simulink model "InnerOuter_Sim"  (Simulink 6.6)
settings: Solver=ode4  StartTime=0.0  StopTime=700  FixedStep=SampleT  RelTol=1e-3
InitFcn:
  | clc
  | Rascal_Var
  | innerOuterInit
  | wpFile
values from neighbouring files (symbols this model uses):
  A1 = 0.007    [Rascal_Var.m]
  Apolar = 0.057    [Rascal_Var.m]
  apSampleTime = 0.01    [innerOuterInit.m]
  CD0 = 0.022    [Rascal_Var.m]
  chord = S/span    (= 0.351341681574)    [Rascal_Var.m]
  CL0 = 0.38    [Rascal_Var.m]
  CLa = 18.5    [Rascal_Var.m]
  CLa_dot = 2.64    [Rascal_Var.m]
  Clb = -0.296    [Rascal_Var.m]
  ClDa = 0.1695    [Rascal_Var.m]
  CLDe = 0.24    [Rascal_Var.m]
  CLDf = 0.4    [Rascal_Var.m]
  ClDr = 0.106    [Rascal_Var.m]
  Clp = -1.96    [Rascal_Var.m]
  CLq = 7.4    [Rascal_Var.m]
  Clr = 0.103    [Rascal_Var.m]
  Cm0 = 0.3    [Rascal_Var.m]
  Cma = -1.239    [Rascal_Var.m]
  CmDe = -3.2    [Rascal_Var.m]
  CmDf = -.021    (= -0.021)    [Rascal_Var.m]
  Cmq = -2.4    [Rascal_Var.m]
  Cnb = 0.277    [Rascal_Var.m]
  CnDa = -0.023    [Rascal_Var.m]
  CnDr = -0.1997    [Rascal_Var.m]
  Cnp = -0.0889    [Rascal_Var.m]
  Cnr = -0.19997    [Rascal_Var.m]
  CYb = -1.098    [Rascal_Var.m]
  CYDr = 0.143    [Rascal_Var.m]
  derivativesConstant = 5    [innerOuterInit.m]
  elarm = 1.21    [Rascal_Var.m]
  Euler_0 = [0; 0; 90*pi/180]'    [Rascal_Var.m]    (also in randomInit.m = double([0; 0; psi_ic]'))
  ISA_g = 9.815    [Rascal_Var.m]
  Ixx = 4.12    [Rascal_Var.m]
  Iyy = 9.58    [Rascal_Var.m]
  Izz = 9.85    [Rascal_Var.m]
  mass = 0.45359237*18    (= 8.16466266)    [Rascal_Var.m]
  MinThK = 0.077    [Rascal_Var.m]
  Pos_0 = [0; 0 ;450]'    [Rascal_Var.m]    (also in randomInit.m = double([x_ic y_ic z_ic]))
  PQR_0 = [0;0;0]'    [Rascal_Var.m]
  SampleT = 0.005    [Rascal_Var.m]    (also in innerOuterInit.m)
  span = 2.795    [Rascal_Var.m]
  ThK = 2.17    [Rascal_Var.m]
  Vb_0 = [ 25; 0;0]'    [Rascal_Var.m]
  wpCount = uint8(floor(getRanVal(7,4,10)))    [randomInit.m]
undefined symbols (not defined in the file or in its folder): bankCommandLimit, clock, daLimit, deg, deLimit, DiscIntNeverNeededParam, drLimit, dtLimit, Earth, heightErrorLimit, pitchCommandLimit, pitchErrorLimit, rad, rollControlLimit, s, uHoldLimit, WGS84, yawDamperLimit
libraries: simulink x54, SLUGS_Library x14, aerolibconvert2 x9, aerolibtransform2 x2, aerolibwind2 x1, aerolibatmos2 x1, dspmtrx3 x1, dsPICdrivers x1
(part 2 of 2)

== system InnerOuter_Sim/6DOF Model/Plant/Engine Model/Get To1 ==
  dt : Inport
  Divide : Product  Inputs=3  OutScaling=2^-10
  Math Function : Math  Operator=pow  SaturateOnIntegerOverflow=on
  Math Function1 : Math  Operator=pow  SaturateOnIntegerOverflow=on
  MaxRPM : Gain  Gain=7200  SaturateOnIntegerOverflow=on
  Min RPM : Constant  Value=2000
  Min Th K : Constant  Value=MinThK
  Prop Diameter (in) : Constant  Value=17
  Prop Diameter (in)1 : Constant  Value=2
  Prop Diameter (in)2 : Constant  Value=4
  Saturation : Saturate  UpperLimit=1.0  LowerLimit=0.2
  Sum : Sum  Inputs=|++
  Sum1 : Sum  Inputs=|++
  TFact : simulink/Math Operations/Slider Gain  SystemSampleTime=-1  low=0  gain=0.2  high=1
  Th K : Gain  Gain=ThK  SaturateOnIntegerOverflow=on
  To Constant : Constant  Value=2.83e-12
  To : Outport
  wires:
  Saturation/1 -> Th K/1
  Prop Diameter (in)1/1 -> Math Function/2
  Prop Diameter (in)2/1 -> Math Function1/2
  Prop Diameter (in)/1 -> Math Function1/1
  Math Function/1 -> Divide/1
  Math Function1/1 -> Divide/2
  To Constant/1 -> Divide/3
  Divide/1 -> TFact/1
  TFact/1 -> To/1
  Sum/1 -> Math Function/1
  Min RPM/1 -> Sum/2
  MaxRPM/1 -> Sum/1
  Th K/1 -> Sum1/1
  dt/1 -> Saturation/1
  Sum1/1 -> MaxRPM/1
  Min Th K/1 -> Sum1/2

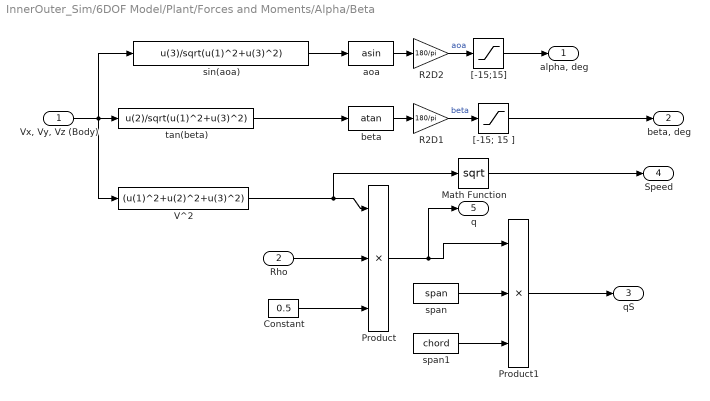
== system InnerOuter_Sim/6DOF Model/Plant/Forces and Moments/Alpha/Beta ==
  "Vx, Vy, Vz (Body)" : Inport
  Rho : Inport  Port=2
  Constant : Constant  Value=0.5  VectorParams1D=off
  Math Function : Math  Operator=sqrt  SaturateOnIntegerOverflow=on
  Product : Product  Inputs=3  SaturateOnIntegerOverflow=on
  Product1 : Product  Inputs=3  SaturateOnIntegerOverflow=on
  R2D1 : Gain  Gain=180/pi  SaturateOnIntegerOverflow=on
  R2D2 : Gain  Gain=180/pi  SaturateOnIntegerOverflow=on
  V^2 : Fcn  Expr=(u(1)^2+u(2)^2+u(3)^2)
  "[-15; 15 ]" : Saturate  UpperLimit=15  LowerLimit=-15
  "[-15;15]" : Saturate  UpperLimit=15  LowerLimit=-15
  aoa : Trigonometry  Operator=asin
  beta : Trigonometry  Operator=atan
  sin(aoa) : Fcn  Expr=u(3)/sqrt(u(1)^2+u(3)^2)
  span : Constant  Value=span  VectorParams1D=off
  span1 : Constant  Value=chord  VectorParams1D=off
  tan(beta) : Fcn  Expr=u(2)/sqrt(u(1)^2+u(3)^2)
  "alpha, deg" : Outport
  "beta, deg" : Outport  Port=2
  qS : Outport  Port=3
  Speed : Outport  Port=4
  q : Outport  Port=5
  wires:
  Product/1 -> q/1, Product1/1
  Product1/1 -> qS/1
  span1/1 -> Product1/3
  span/1 -> Product1/2
  "Vx, Vy, Vz (Body)"/1 -> sin(aoa)/1, V^2/1, tan(beta)/1
  tan(beta)/1 -> beta/1
  beta/1 -> R2D1/1
  V^2/1 -> Product/1, Math Function/1
  Rho/1 -> Product/2
  Constant/1 -> Product/3
  R2D1/1 -> "[-15; 15 ]"/1  "beta"
  aoa/1 -> R2D2/1
  R2D2/1 -> "[-15;15]"/1  "aoa"
  sin(aoa)/1 -> aoa/1
  Math Function/1 -> Speed/1
  "[-15;15]"/1 -> "alpha, deg"/1
  "[-15; 15 ]"/1 -> "beta, deg"/1

== system InnerOuter_Sim/6DOF Model/Plant/Forces and Moments/Body Frame F & M ==
  "Alpha, deg" : Inport
  "Beta, deg" : Inport  Port=2
  qs : Inport  Port=3
  Airspeed : Inport  Port=4
  "de, deg" : Inport  Port=5
  "da, deg" : Inport  Port=6
  "dr, deg" : Inport  Port=7
  "df, deg" : Inport  Port=8
  p,q,r : Inport  Port=9
  Bus Creator : BusCreator  Inputs=2
  Transfer to body frame : Subsystem
  Wind frame F& M : Subsystem
  F_b : Outport
  M_b : Outport  Port=2
  wires:
  "Alpha, deg"/1 -> Wind frame F& M/1("alpha, deg"), Bus Creator/1
  "Beta, deg"/1 -> Wind frame F& M/2("beta, deg"), Bus Creator/2
  "dr, deg"/1 -> Wind frame F& M/5("dr, deg")
  "da, deg"/1 -> Wind frame F& M/4("da, deg")
  "de, deg"/1 -> Wind frame F& M/3("de, deg")
  Wind frame F& M/1(F&M wind frame) -> Transfer to body frame/1(Wind frame  F&M)
  Bus Creator/1 -> Transfer to body frame/2("aoa/beta, deg")  "aoa/beta, deg"
  Transfer to body frame/1(F_b) -> F_b/1
  Transfer to body frame/2(M_b) -> M_b/1
  "df, deg"/1 -> Wind frame F& M/6("df, deg")
  qs/1 -> Wind frame F& M/7(qS)
  p,q,r/1 -> Wind frame F& M/8(p,q,r)
  Airspeed/1 -> Wind frame F& M/9(Airpseed)

== system InnerOuter_Sim/6DOF Model/Plant/Forces and Moments/Get Grav Force in Body ==
  Euler : Inport
  Grav Force : Inport  Port=2
  Math Function : Math  Operator=transpose  SaturateOnIntegerOverflow=on
  Product1 : Product  Multiplication=Matrix(*)  SaturateOnIntegerOverflow=on  InputSameDT=on
  Rb2u : Subsystem
  Reshape : Reshape  OutputDimensionality=Column vector (2-D)
  Grav Force (Body) : Outport
  wires:
  Rb2u/1(DCM) -> Math Function/1
  Euler/1 -> Rb2u/1(phi theta psi)
  Product1/1 -> Grav Force (Body)/1
  Math Function/1 -> Product1/1
  Grav Force/1 -> Reshape/1
  Reshape/1 -> Product1/2

== system InnerOuter_Sim/6DOF Model/Plant/Forces and Moments/NED(u)2b ==
  V w : Inport
  Euler : Inport  Port=2
  RB2LTP : Subsystem
  RL2B * Vw : Product  Multiplication=Matrix(*)  SaturateOnIntegerOverflow=on  InputSameDT=on
  RLTP2B : Math  Operator=transpose  SaturateOnIntegerOverflow=on
  Reshape1 : Reshape  OutputDimensionality=Row vector (2-D)
  Vb Corr : Outport
  wires:
  RL2B * Vw/1 -> Reshape1/1
  Euler/1 -> RB2LTP/1(Euler)
  RB2LTP/1(RB2L) -> RLTP2B/1
  RLTP2B/1 -> RL2B * Vw/1
  V w/1 -> RL2B * Vw/2
  Reshape1/1 -> Vb Corr/1

== system InnerOuter_Sim/6DOF Model/Plant/Magnetometer/RB2LTP ==
  Euler : Inport
  11 : Fcn  Expr=cos(u[3])*cos(u[2])
  12 : Fcn  Expr=sin(u[3])*cos(u[2])
  13 : Fcn  Expr=-sin(u[2])
  21 : Fcn  Expr=cos(u[3])*sin(u[2])*sin(u[1])-sin(u[3])*cos(u[1])
  22 : Fcn  Expr=sin(u[3])*sin(u[2])*sin(u[1])+cos(u[3])*cos(u[1])
  23 : Fcn  Expr=cos(u[2])*sin(u[1])
  31 : Fcn  Expr=cos(u[3])*sin(u[2])*cos(u[1])+sin(u[3])*sin(u[1])
  32 : Fcn  Expr=sin(u[3])*sin(u[2])*cos(u[1])-cos(u[3])*sin(u[1])
  33 : Fcn  Expr=cos(u[2])*cos(u[1])
  Mux2 : Mux  Inputs=9
  Reshape : Reshape  OutputDimensionality=Customize  OutputDimensions=[3,3]
  Rot : Outport
  wires:
  33/1 -> Mux2/9
  32/1 -> Mux2/8
  31/1 -> Mux2/7
  23/1 -> Mux2/6
  22/1 -> Mux2/5
  21/1 -> Mux2/4
  13/1 -> Mux2/3
  12/1 -> Mux2/2
  11/1 -> Mux2/1
  Mux2/1 -> Reshape/1
  Euler/1 -> 11/1, 33/1, 32/1, 31/1, 23/1, 22/1, 21/1, 13/1, 12/1
  Reshape/1 -> Rot/1

== system InnerOuter_Sim/6DOF Model/Plant/Wrap Around PSI1/Negative Yaw ==
  yaw : Inport
  Enable : EnablePort
  Abs : Abs
  Constant1 : Constant  Value=2*pi
  Constant2 : Constant  Value=2*pi
  Math Function : Math  Operator=mod  SaturateOnIntegerOverflow=on
  Sum : Sum  Inputs=|-+
  yaw_wr : Outport
  wires:
  yaw/1 -> Abs/1
  Constant1/1 -> Math Function/2
  Math Function/1 -> Sum/1
  Abs/1 -> Math Function/1
  Constant2/1 -> Sum/2
  Sum/1 -> yaw_wr/1

== system InnerOuter_Sim/6DOF Model/Plant/Wrap Around PSI1/Positive Yaw ==
  yaw : Inport
  Enable : EnablePort
  Constant1 : Constant  Value=2*pi
  Math Function : Math  Operator=mod  SaturateOnIntegerOverflow=on
  yaw_wr : Outport
  wires:
  yaw/1 -> Math Function/1
  Constant1/1 -> Math Function/2
  Math Function/1 -> yaw_wr/1

== system InnerOuter_Sim/6DOF Model/Plant/6-DOF EOM/[V1,2,3,W1,2,3]/A = [M ; J] ==
  Constant1 : Constant  Value=zeros(3,3)
  Constant4 : Constant  Value=0
  Display : Display
  Display1 : Display
  Display2 : Display
  Ixx : Constant  Value=Ixx  VectorParams1D=off
  Iyy : Constant  Value=Iyy  VectorParams1D=off
  Izz : Constant  Value=Izz  VectorParams1D=off
  Matrix Concatenation : Concatenate  Mode=Multidimensional array
  Matrix Concatenation1 : Concatenate  Mode=Multidimensional array
  Matrix Concatenation2 : Concatenate  Mode=Multidimensional array  ConcatenateDimension=2
  Mux : Mux  Inputs=9
  Mux1 : Mux  Inputs=9
  Reshape : Reshape  OutputDimensionality=Customize  OutputDimensions=[3,3]
  Reshape1 : Reshape  OutputDimensionality=Customize  OutputDimensions=[3,3]
  mass : Constant  Value=mass  VectorParams1D=off
  A Matrix : Outport
  wires:
  Ixx/1 -> Mux/1
  Izz/1 -> Mux/9
  Iyy/1 -> Mux/5
  Constant4/1 -> Mux/8, Mux/7, Mux/6, Mux/4, Mux/3, Mux/2, Mux1/8, Mux1/7, Mux1/6, Mux1/4, Mux1/3, Mux1/2
  mass/1 -> Mux1/1, Mux1/5, Mux1/9
  Mux1/1 -> Reshape/1
  Mux/1 -> Reshape1/1
  Matrix Concatenation/1 -> Matrix Concatenation2/1, Display/1
  Matrix Concatenation1/1 -> Matrix Concatenation2/2, Display1/1
  Matrix Concatenation2/1 -> A Matrix/1, Display2/1
  Reshape1/1 -> Matrix Concatenation1/2
  Reshape/1 -> Matrix Concatenation/1
  Constant1/1 -> Matrix Concatenation/2, Matrix Concatenation1/1

== system InnerOuter_Sim/6DOF Model/Plant/6-DOF EOM/[V1,2,3,W1,2,3]/Get Grav Force in Body ==
  Euler : Inport
  Grav Force : Inport  Port=2
  Math Function : Math  Operator=transpose  SaturateOnIntegerOverflow=on
  Product1 : Product  Multiplication=Matrix(*)  SaturateOnIntegerOverflow=on  InputSameDT=on
  Rb2u : Subsystem
  Reshape : Reshape  OutputDimensionality=Column vector (2-D)
  Grav Force (Body) : Outport
  wires:
  Rb2u/1(DCM) -> Math Function/1
  Euler/1 -> Rb2u/1(phi theta psi)
  Product1/1 -> Grav Force (Body)/1
  Math Function/1 -> Product1/1
  Grav Force/1 -> Reshape/1
  Reshape/1 -> Product1/2

== system InnerOuter_Sim/6DOF Model/Plant/6-DOF EOM/[V1,2,3,W1,2,3]/Sigma ==
  note: S(pqr)
  pqr : Inport
  Gain : Gain  Gain=[0 0 0;0 0 -1; 0 1 0]  Multiplication=Matrix(K*u)  SaturateOnIntegerOverflow=on
  Gain1 : Gain  Gain=[0 0 1;0 0 0; -1 0 0]  Multiplication=Matrix(K*u)  SaturateOnIntegerOverflow=on
  Gain2 : Gain  Gain="[0 -1 0;1 0 0;  0 0 0]"  Multiplication=Matrix(K*u)  SaturateOnIntegerOverflow=on
  Gain3 : Gain  Gain=0  SaturateOnIntegerOverflow=on
  Math Function : Math  Operator=transpose  SaturateOnIntegerOverflow=on
  Matrix Concatenation : Concatenate  Mode=Multidimensional array  ConcatenateDimension=2
  Matrix Concatenation1 : Concatenate  Mode=Multidimensional array  ConcatenateDimension=2
  Matrix Concatenation2 : Concatenate  Mode=Multidimensional array
  Mux : Mux  Inputs=3
  Reshape : Reshape  OutputDimensionality=Customize  OutputDimensions=[3,3]
  Sigma : Outport
  wires:
  Mux/1 -> Reshape/1
  Gain/1 -> Mux/1
  Gain1/1 -> Mux/2
  Gain2/1 -> Mux/3
  Reshape/1 -> Math Function/1
  Math Function/1 -> Gain3/1, Matrix Concatenation/1, Matrix Concatenation1/2
  Gain3/1 -> Matrix Concatenation/2, Matrix Concatenation1/1
  Matrix Concatenation/1 -> Matrix Concatenation2/1
  Matrix Concatenation1/1 -> Matrix Concatenation2/2
  Matrix Concatenation2/1 -> Sigma/1
  pqr/1 -> Gain/1, Gain2/1, Gain1/1

== system InnerOuter_Sim/6DOF Model/Plant/Forces and Moments/Body Frame F & M/Transfer to body frame ==
  Wind frame  F&M : Inport
  "aoa/beta, deg" : Inport  Port=2
  D2R : Gain  Gain=pi/180  SaturateOnIntegerOverflow=on
  Forces : Selector  IndexOptions=Index vector (dialog)  Indices=[1 2 3]  OutputSizes=[(-2)]  InputPortWidth=6
  Moments : Selector  IndexOptions=Index vector (dialog)  Indices=[4 5 6]  OutputSizes=[(-2)]  InputPortWidth=6
  Ra2b1 : Subsystem
  Ra2b22 : Subsystem
  Scope : Scope
      settings: YMin=-450  YMax=200  SaveName=ScopeData11
  Scope1 : Scope
      settings: YMin=-450  YMax=200  SaveName=ScopeData17
  F_b : Outport
  M_b : Outport  Port=2
  wires:
  Ra2b1/1(body frame) -> F_b/1, Scope/1  "Fb"
  Ra2b22/1(body frame) -> Scope1/1, M_b/1  "Mb"
  "aoa/beta, deg"/1 -> D2R/1
  Forces/1 -> Ra2b1/1(wind frame)
  Wind frame  F&M/1 -> Forces/1, Moments/1
  Moments/1 -> Ra2b22/2(wind frame)
  D2R/1 -> Ra2b1/2(aoa/beta), Ra2b22/1(aoa/beta)

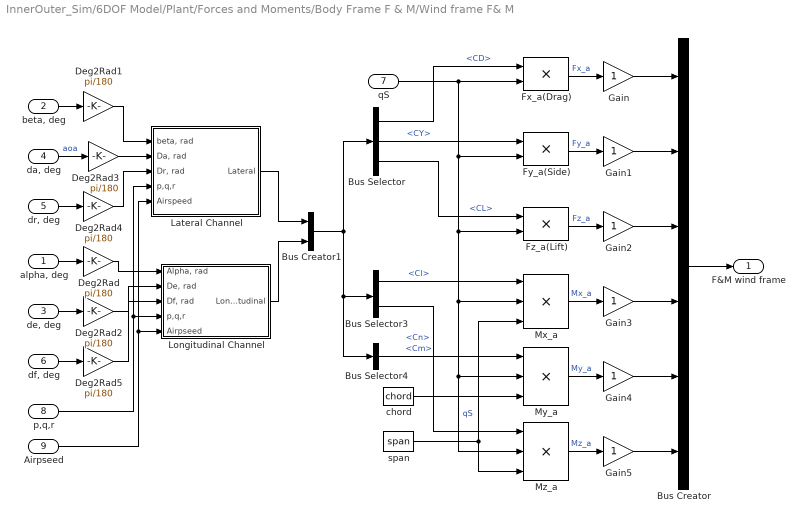
== system InnerOuter_Sim/6DOF Model/Plant/Forces and Moments/Body Frame F & M/Wind frame F& M ==
  "alpha, deg" : Inport
  "beta, deg" : Inport  Port=2
  "de, deg" : Inport  Port=3
  "da, deg" : Inport  Port=4
  "dr, deg" : Inport  Port=5
  "df, deg" : Inport  Port=6
  qS : Inport  Port=7
  p,q,r : Inport  Port=8
  Airpseed : Inport  Port=9
  Bus Creator : BusCreator  Inputs=6
  Bus Creator1 : BusCreator  Inputs=2
  Bus Selector : BusSelector  OutputSignals=signal2.CD,signal1.CY,signal2.CL
  Bus Selector3 : BusSelector  OutputSignals=signal1.Cl,signal1.Cn
  Bus Selector4 : BusSelector  OutputSignals=signal2.Cm
  Deg2Rad{,1..5} (6 alike) : Gain  Gain=pi/180  SaturateOnIntegerOverflow=on
  Fx_a(Drag) : Product  Inputs=**  SaturateOnIntegerOverflow=on
  Fy_a(Side) : Product  SaturateOnIntegerOverflow=on
  Fz_a(Lift) : Product  SaturateOnIntegerOverflow=on
  Gain{,1..5} (6 alike) : Gain  SaturateOnIntegerOverflow=on
  Lateral Channel : Subsystem
  Longitudinal Channel : Subsystem
  Mx_a : Product  Inputs=3  SaturateOnIntegerOverflow=on
  My_a : Product  Inputs=3  SaturateOnIntegerOverflow=on
  Mz_a : Product  Inputs=3  SaturateOnIntegerOverflow=on
  chord : Constant  Value=chord  VectorParams1D=off
  span : Constant  Value=span  VectorParams1D=off
  F&M wind frame : Outport
  wires:
  Bus Selector/1 -> Fx_a(Drag)/1  "<CD>"
  Fx_a(Drag)/1 -> Gain/1  "Fx_a"
  Fy_a(Side)/1 -> Gain1/1  "Fy_a"
  Fz_a(Lift)/1 -> Gain2/1  "Fz_a"
  Bus Selector3/1 -> Mx_a/1  "<Cl>"
  Mx_a/1 -> Gain3/1  "Mx_a"
  Bus Selector4/1 -> My_a/1  "<Cm>"
  Mz_a/1 -> Gain5/1  "Mz_a"
  qS/1 -> Fx_a(Drag)/2, Fy_a(Side)/2, Fz_a(Lift)/2, Mx_a/2, My_a/2, Mz_a/2  "qS"
  span/1 -> Mx_a/3, Mz_a/3
  chord/1 -> My_a/3
  Bus Selector/2 -> Fy_a(Side)/1  "<CY>"
  Bus Selector/3 -> Fz_a(Lift)/1  "<CL>"
  Bus Selector3/2 -> Mz_a/1  "<Cn>"
  Bus Creator/1 -> F&M wind frame/1
  My_a/1 -> Gain4/1  "My_a"
  Bus Creator1/1 -> Bus Selector/1, Bus Selector3/1, Bus Selector4/1
  Longitudinal Channel/1(Longitudinal) -> Bus Creator1/2
  "alpha, deg"/1 -> Deg2Rad/1
  "beta, deg"/1 -> Deg2Rad1/1
  "de, deg"/1 -> Deg2Rad2/1
  "da, deg"/1 -> Deg2Rad3/1  "aoa"
  "dr, deg"/1 -> Deg2Rad4/1
  Deg2Rad1/1 -> Lateral Channel/1("beta, rad")
  Deg2Rad4/1 -> Lateral Channel/3("Dr, rad")
  Deg2Rad/1 -> Longitudinal Channel/1("Alpha, rad")
  Deg2Rad2/1 -> Longitudinal Channel/2("De, rad")
  Gain/1 -> Bus Creator/1
  Gain1/1 -> Bus Creator/2
  Gain2/1 -> Bus Creator/3
  Gain3/1 -> Bus Creator/4
  Gain4/1 -> Bus Creator/5
  Gain5/1 -> Bus Creator/6
  "df, deg"/1 -> Deg2Rad5/1
  Deg2Rad5/1 -> Longitudinal Channel/3("Df, rad")
  Lateral Channel/1(Lateral) -> Bus Creator1/1
  p,q,r/1 -> Lateral Channel/4(p,q,r), Longitudinal Channel/4(p,q,r)
  Airpseed/1 -> Lateral Channel/5(Airspeed), Longitudinal Channel/5(Airpseed)
  Deg2Rad3/1 -> Lateral Channel/2("Da, rad")

== system InnerOuter_Sim/6DOF Model/Plant/Forces and Moments/Get Grav Force in Body/Rb2u ==
  phi theta psi : Inport
  11 : Fcn  Expr=cos(u[3])*cos(u[2])
  12 : Fcn  Expr=sin(u[3])*cos(u[2])
  13 : Fcn  Expr=-sin(u[2])
  21 : Fcn  Expr=cos(u[3])*sin(u[2])*sin(u[1])-sin(u[3])*cos(u[1])
  22 : Fcn  Expr=sin(u[3])*sin(u[2])*sin(u[1])+cos(u[3])*cos(u[1])
  23 : Fcn  Expr=cos(u[2])*sin(u[1])
  31 : Fcn  Expr=cos(u[3])*sin(u[2])*cos(u[1])+sin(u[3])*sin(u[1])
  32 : Fcn  Expr=sin(u[3])*sin(u[2])*cos(u[1])-cos(u[3])*sin(u[1])
  33 : Fcn  Expr=cos(u[2])*cos(u[1])
  Mux2 : Mux  Inputs=9
  Reshape : Reshape  OutputDimensionality=Customize  OutputDimensions=[3,3]
  DCM : Outport  InitialOutput=0
  wires:
  Reshape/1 -> DCM/1
  phi theta psi/1 -> 12/1, 13/1, 21/1, 22/1, 23/1, 31/1, 32/1, 33/1, 11/1
  Mux2/1 -> Reshape/1
  11/1 -> Mux2/1
  12/1 -> Mux2/2
  13/1 -> Mux2/3
  21/1 -> Mux2/4
  22/1 -> Mux2/5
  23/1 -> Mux2/6
  31/1 -> Mux2/7
  32/1 -> Mux2/8
  33/1 -> Mux2/9

== system InnerOuter_Sim/6DOF Model/Plant/Forces and Moments/NED(u)2b/RB2LTP ==
  Euler : Inport
  11 : Fcn  Expr=cos(u[3])*cos(u[2])
  12 : Fcn  Expr=sin(u[3])*cos(u[2])
  13 : Fcn  Expr=-sin(u[2])
  21 : Fcn  Expr=cos(u[3])*sin(u[2])*sin(u[1])-sin(u[3])*cos(u[1])
  22 : Fcn  Expr=sin(u[3])*sin(u[2])*sin(u[1])+cos(u[3])*cos(u[1])
  23 : Fcn  Expr=cos(u[2])*sin(u[1])
  31 : Fcn  Expr=cos(u[3])*sin(u[2])*cos(u[1])+sin(u[3])*sin(u[1])
  32 : Fcn  Expr=sin(u[3])*sin(u[2])*cos(u[1])-cos(u[3])*sin(u[1])
  33 : Fcn  Expr=cos(u[2])*cos(u[1])
  Mux2 : Mux  Inputs=9
  Reshape : Reshape  OutputDimensionality=Customize  OutputDimensions=[3,3]
  RB2L : Outport  InitialOutput=0
  wires:
  33/1 -> Mux2/9
  32/1 -> Mux2/8
  31/1 -> Mux2/7
  23/1 -> Mux2/6
  22/1 -> Mux2/5
  21/1 -> Mux2/4
  13/1 -> Mux2/3
  12/1 -> Mux2/2
  11/1 -> Mux2/1
  Mux2/1 -> Reshape/1
  Euler/1 -> 11/1, 33/1, 32/1, 31/1, 23/1, 22/1, 21/1, 13/1, 12/1
  Reshape/1 -> RB2L/1

== system InnerOuter_Sim/6DOF Model/Plant/6-DOF EOM/[V1,2,3,W1,2,3]/Get Grav Force in Body/Rb2u ==
  phi theta psi : Inport
  11 : Fcn  Expr=cos(u[3])*cos(u[2])
  12 : Fcn  Expr=sin(u[3])*cos(u[2])
  13 : Fcn  Expr=-sin(u[2])
  21 : Fcn  Expr=cos(u[3])*sin(u[2])*sin(u[1])-sin(u[3])*cos(u[1])
  22 : Fcn  Expr=sin(u[3])*sin(u[2])*sin(u[1])+cos(u[3])*cos(u[1])
  23 : Fcn  Expr=cos(u[2])*sin(u[1])
  31 : Fcn  Expr=cos(u[3])*sin(u[2])*cos(u[1])+sin(u[3])*sin(u[1])
  32 : Fcn  Expr=sin(u[3])*sin(u[2])*cos(u[1])-cos(u[3])*sin(u[1])
  33 : Fcn  Expr=cos(u[2])*cos(u[1])
  Mux2 : Mux  Inputs=9
  Reshape : Reshape  OutputDimensionality=Customize  OutputDimensions=[3,3]
  DCM : Outport  InitialOutput=0
  wires:
  Reshape/1 -> DCM/1
  phi theta psi/1 -> 12/1, 13/1, 21/1, 22/1, 23/1, 31/1, 32/1, 33/1, 11/1
  Mux2/1 -> Reshape/1
  11/1 -> Mux2/1
  12/1 -> Mux2/2
  13/1 -> Mux2/3
  21/1 -> Mux2/4
  22/1 -> Mux2/5
  23/1 -> Mux2/6
  31/1 -> Mux2/7
  32/1 -> Mux2/8
  33/1 -> Mux2/9

== system InnerOuter_Sim/6DOF Model/Plant/Forces and Moments/Body Frame F & M/Transfer to body frame/Ra2b1 ==
  wind frame : Inport
  aoa/beta : Inport  Port=2
  Product2 : Product  Multiplication=Matrix(*)  SaturateOnIntegerOverflow=on
  RB2W : Subsystem
  RW2B : Math  Operator=transpose  SaturateOnIntegerOverflow=on
  Reshape : Reshape  OutputDimensionality=Column vector (2-D)
  body frame : Outport
  wires:
  RB2W/1(Rw2b) -> RW2B/1
  aoa/beta/1 -> RB2W/1(aoa beta)
  Product2/1 -> body frame/1
  wind frame/1 -> Reshape/1
  Reshape/1 -> Product2/2
  RW2B/1 -> Product2/1

== system InnerOuter_Sim/6DOF Model/Plant/Forces and Moments/Body Frame F & M/Transfer to body frame/Ra2b22 ==
  aoa/beta : Inport
  wind frame : Inport  Port=2
  Product2 : Product  Multiplication=Matrix(*)  SaturateOnIntegerOverflow=on
  RB2W : Subsystem
  RW2B : Math  Operator=transpose  SaturateOnIntegerOverflow=on
  Reshape : Reshape  OutputDimensionality=Column vector (2-D)
  body frame : Outport
  wires:
  Reshape/1 -> Product2/2
  wind frame/1 -> Reshape/1
  Product2/1 -> body frame/1
  aoa/beta/1 -> RB2W/1(aoa beta)
  RB2W/1(Rw2b) -> RW2B/1
  RW2B/1 -> Product2/1

== system InnerOuter_Sim/6DOF Model/Plant/Forces and Moments/Body Frame F & M/Wind frame F& M/Lateral Channel ==
  "beta, rad" : Inport
  "Da, rad" : Inport  Port=2
  "Dr, rad" : Inport  Port=3
  p,q,r : Inport  Port=4
  Airspeed : Inport  Port=5
  Bus Creator : BusCreator  Inputs=3
  CY : Subsystem
  Cl : Subsystem
  Cn : Subsystem
  Constant : Constant
  Divide : Product  OutScaling=2^-10
  Divide1 : Product  OutScaling=2^-10
  Divide2 : Product  OutScaling=2^-10
  Scope : Scope  NumInputPorts=3
      settings: YMin=-0.035~-0.005~-0.001  YMax=0.015~0.002~0.00125  SaveName=ScopeData7
  Slider Gain : simulink/Math Operations/Slider Gain  SystemSampleTime=-1  low=0  gain=1  high=2
  Lateral : Outport
  wires:
  Divide2/1 -> Bus Creator/3  "Cn"
  Divide1/1 -> Bus Creator/2  "Cl"
  Divide/1 -> Bus Creator/1  "CY"
  Slider Gain/1 -> Divide2/2, Divide1/2, Divide/2
  Constant/1 -> Slider Gain/1
  Bus Creator/1 -> Lateral/1
  CY/1(CY) -> Divide/1, Scope/1  "CY"
  Cl/1(Cl) -> Divide1/1, Scope/2  "Cl"
  Cn/1(Cn) -> Divide2/1, Scope/3  "Cn"
  "beta, rad"/1 -> CY/1(beta), Cl/1(beta), Cn/1(beta)
  "Da, rad"/1 -> Cl/2(Da), Cn/2(Da)
  "Dr, rad"/1 -> Cn/3(Dr), Cl/3(Dr), CY/2(Dr)
  Airspeed/1 -> Cn/5(Airspeed), Cl/5(Airspeed)
  p,q,r/1 -> Cn/4(p,q,r), Cl/4(p,q,r)

== system InnerOuter_Sim/6DOF Model/Plant/Forces and Moments/Body Frame F & M/Wind frame F& M/Longitudinal Channel ==
  "Alpha, rad" : Inport
  "De, rad" : Inport  Port=2
  "Df, rad" : Inport  Port=3
  p,q,r : Inport  Port=4
  Airpseed : Inport  Port=5
  Bus Creator : BusCreator  Inputs=3
  CD : Subsystem
  CL : Subsystem
  Cm : Subsystem
  Gain : Gain  Gain=-1  SaturateOnIntegerOverflow=on
  Transfer Fcn : TransferFcn  Numerator=[1 0]  Denominator=[0.1 1]
  Y-down : Gain  Gain=-1  SaturateOnIntegerOverflow=on
  Longitudinal : Outport
  wires:
  "Alpha, rad"/1 -> CL/1(alpha), Cm/1(alpha), Transfer Fcn/1
  CD/1(CD) -> Gain/1
  Gain/1 -> Bus Creator/1  "CD"
  Y-down/1 -> Bus Creator/2  "CL"
  "De, rad"/1 -> CL/3(De), Cm/2(De)
  CL/1(CL) -> Y-down/1, CD/1(CL)
  Cm/1(Cm) -> Bus Creator/3  "Cm"
  Bus Creator/1 -> Longitudinal/1
  "Df, rad"/1 -> CL/4(Df), Cm/3(Df)
  p,q,r/1 -> CL/5(p,q,r), Cm/4(p,q,r)
  Airpseed/1 -> CL/6(Airspeed)
  Transfer Fcn/1 -> CL/2(alpha_dot)

== system InnerOuter_Sim/6DOF Model/Plant/Forces and Moments/Body Frame F & M/Transfer to body frame/Ra2b1/RB2W ==
  aoa beta : Inport
  11 : Fcn  Expr=cos(u[1])*cos(u[2])
  12 : Fcn  Expr=sin(u[2])
  13 : Fcn  Expr=sin(u[1])*cos(u[2])
  21 : Fcn  Expr=-cos(u[1])*sin(u[2])
  22 : Fcn  Expr=cos(u[2])
  23 : Fcn  Expr=-sin(u[1])*sin(u[2])
  31 : Fcn  Expr=-sin(u[1])
  32 : Fcn  Expr=0
  33 : Fcn  Expr=cos(u[1])
  Mux3 : Mux  Inputs=9
  Reshape 9x1->3x3 : Reshape  OutputDimensionality=Customize  OutputDimensions=[3,3]
  Rw2b : Outport  InitialOutput=0
  wires:
  aoa beta/1 -> 11/1, 21/1, 31/1, 12/1, 22/1, 32/1, 13/1, 23/1, 33/1
  Mux3/1 -> Reshape 9x1->3x3/1
  Reshape 9x1->3x3/1 -> Rw2b/1
  11/1 -> Mux3/1
  21/1 -> Mux3/2
  31/1 -> Mux3/3
  12/1 -> Mux3/4
  22/1 -> Mux3/5
  32/1 -> Mux3/6
  13/1 -> Mux3/7
  23/1 -> Mux3/8
  33/1 -> Mux3/9

== system InnerOuter_Sim/6DOF Model/Plant/Forces and Moments/Body Frame F & M/Transfer to body frame/Ra2b22/RB2W ==
  aoa beta : Inport
  11 : Fcn  Expr=cos(u[1]) * cos(u[2])
  12 : Fcn  Expr=sin(u[2])
  13 : Fcn  Expr=sin(u[1]) * cos(u[2])
  21 : Fcn  Expr=-cos(u[1]) * sin(u[2])
  22 : Fcn  Expr=cos(u[2])
  23 : Fcn  Expr=-sin(u[1]) * sin(u[2])
  31 : Fcn  Expr=-sin(u[1])
  32 : Fcn  Expr=0
  33 : Fcn  Expr=cos(u[1])
  Mux3 : Mux  Inputs=9
  Reshape 9x1->3x3 : Reshape  OutputDimensionality=Customize  OutputDimensions=[3,3]
  Rw2b : Outport  InitialOutput=0
  wires:
  33/1 -> Mux3/9
  23/1 -> Mux3/8
  13/1 -> Mux3/7
  32/1 -> Mux3/6
  22/1 -> Mux3/5
  12/1 -> Mux3/4
  31/1 -> Mux3/3
  21/1 -> Mux3/2
  11/1 -> Mux3/1
  Reshape 9x1->3x3/1 -> Rw2b/1
  Mux3/1 -> Reshape 9x1->3x3/1
  aoa beta/1 -> 33/1, 23/1, 13/1, 32/1, 22/1, 12/1, 31/1, 21/1, 11/1

== system InnerOuter_Sim/6DOF Model/Plant/Forces and Moments/Body Frame F & M/Wind frame F& M/Lateral Channel/CY ==
  beta : Inport
  Dr : Inport  Port=2
  CYDr : Constant  Value=CYDr
  "CYDr " : simulink/Math Operations/Slider Gain  SystemSampleTime=-1  low=-2  gain=1  high=2
  CYb : Constant  Value=CYb
  "CYb " : simulink/Math Operations/Slider Gain  SystemSampleTime=-1  low=0  gain=1  high=2
  Product : Product  SaturateOnIntegerOverflow=on
  Product1 : Product  SaturateOnIntegerOverflow=on
  Sum2 : Sum  SaturateOnIntegerOverflow=on
  CY : Outport
  wires:
  CYb/1 -> Product/1
  Product/1 -> "CYb "/1
  beta/1 -> Product/2
  Sum2/1 -> CY/1
  "CYb "/1 -> Sum2/1
  CYDr/1 -> Product1/1
  Product1/1 -> "CYDr "/1
  Dr/1 -> Product1/2
  "CYDr "/1 -> Sum2/2

== system InnerOuter_Sim/6DOF Model/Plant/Forces and Moments/Body Frame F & M/Wind frame F& M/Lateral Channel/Cl ==
  beta : Inport
  Da : Inport  Port=2
  Dr : Inport  Port=3
  p,q,r : Inport  Port=4
  Airspeed : Inport  Port=5
  ClDa : Constant  Value=ClDa
  ClDr : Constant  Value=ClDr
  Clb : Constant  Value=Clb
  "Clb " : simulink/Math Operations/Slider Gain  SystemSampleTime=-1  low=-5  gain=1  high=5
  "Clda " : simulink/Math Operations/Slider Gain  SystemSampleTime=-1  low=-120  gain=1  high=120
  Cldr : simulink/Math Operations/Slider Gain  SystemSampleTime=-1  low=-60  gain=1  high=120
  Product1 : Product  SaturateOnIntegerOverflow=on
  Product4 : Product  SaturateOnIntegerOverflow=on
  Product5 : Product  SaturateOnIntegerOverflow=on
  Scope : Scope  NumInputPorts=5
      settings: TickLabels=on  YMin=-0.003~-0.0075~-0.000175~-0.06~-0.04  YMax=0.0015~0.0075~7.5e-005~0.04~0.06  SaveName=ScopeData18
  Sum : Sum  Inputs=+++++  SaturateOnIntegerOverflow=on
  roll factors : Subsystem
  Cl : Outport
  wires:
  Clb/1 -> Product4/1
  Product4/1 -> "Clb "/1
  beta/1 -> Product4/2  "betta"
  ClDa/1 -> Product5/1
  Product5/1 -> "Clda "/1
  Da/1 -> Product5/2  "ail"
  ClDr/1 -> Product1/1
  Product1/1 -> Cldr/1
  Dr/1 -> Product1/2  "dr"
  Sum/1 -> Cl/1
  "Clb "/1 -> Scope/1, Sum/1  "Clb"
  "Clda "/1 -> Scope/2, Sum/2  "Clda"
  Cldr/1 -> Scope/3, Sum/3  "Cldr"
  roll factors/2(Clr) -> Scope/5, Sum/5
  roll factors/1(Clp) -> Scope/4, Sum/4
  p,q,r/1 -> roll factors/1(p,q,r)
  Airspeed/1 -> roll factors/2(Airspeed)

== system InnerOuter_Sim/6DOF Model/Plant/Forces and Moments/Body Frame F & M/Wind frame F& M/Lateral Channel/Cn ==
  beta : Inport
  Da : Inport  Port=2
  Dr : Inport  Port=3
  p,q,r : Inport  Port=4
  Airspeed : Inport  Port=5
  CnDa : Constant  Value=CnDa
  CnDr : Constant  Value=CnDr
  Cnb : Constant  Value=Cnb
  Product1 : Product  SaturateOnIntegerOverflow=on
  Product4 : Product  SaturateOnIntegerOverflow=on
  Product5 : Product  SaturateOnIntegerOverflow=on
  Scope : Scope  NumInputPorts=5
      settings: TickLabels=on  YMin=-0.003~-0.00125~-0.00125~-0.0002~-0.0005  YMax=0.005~0.00125~0.0005~0.0002~0.0005  SaveName=ScopeData4
  Sum : Sum  Inputs=+++++  SaturateOnIntegerOverflow=on
  "tune CnDa " : simulink/Math Operations/Slider Gain  SystemSampleTime=-1  low=0  gain=1  high=100
  "tune CnDr " : simulink/Math Operations/Slider Gain  SystemSampleTime=-1  low=0  gain=1  high=2
  tune Cnb : simulink/Math Operations/Slider Gain  SystemSampleTime=-1  low=-2  gain=1  high=20
  yaw factors : Subsystem
  Cn : Outport
  wires:
  tune Cnb/1 -> Scope/1, Sum/1
  yaw factors/1(Cnp) -> Scope/4, Sum/4
  yaw factors/2(Cnr) -> Scope/5, Sum/5
  "tune CnDr "/1 -> Scope/3, Sum/3
  "tune CnDa "/1 -> Scope/2, Sum/2
  Sum/1 -> Cn/1
  Dr/1 -> Product1/2
  Product1/1 -> "tune CnDr "/1
  CnDr/1 -> Product1/1
  Da/1 -> Product5/2
  Product5/1 -> "tune CnDa "/1
  CnDa/1 -> Product5/1
  beta/1 -> Product4/2
  Product4/1 -> tune Cnb/1
  Cnb/1 -> Product4/1
  p,q,r/1 -> yaw factors/1(p,q,r)
  Airspeed/1 -> yaw factors/2(Airspeed)

== system InnerOuter_Sim/6DOF Model/Plant/Forces and Moments/Body Frame F & M/Wind frame F& M/Longitudinal Channel/CD ==
  CL : Inport
  Apolar : Constant  Value=A1
  Apolar (A2) : Constant  Value=Apolar
  CD0 : Constant  Value=CD0
  Math Function : Math  Operator=square  SaturateOnIntegerOverflow=on
  Product : Product  SaturateOnIntegerOverflow=on
  Product1 : Product  SaturateOnIntegerOverflow=on
  Sum1 : Sum  Inputs=+++  SaturateOnIntegerOverflow=on
  "tune A1 " : simulink/Math Operations/Slider Gain  SystemSampleTime=-1  low=0  gain=1  high=2
  tune APolar : simulink/Math Operations/Slider Gain  SystemSampleTime=-1  low=0  gain=1  high=2
  tune CD0 : simulink/Math Operations/Slider Gain  SystemSampleTime=-1  low=0  gain=1  high=2
  CD : Outport
  wires:
  "tune A1 "/1 -> Product1/2
  tune CD0/1 -> Sum1/1
  Sum1/1 -> CD/1
  CD0/1 -> tune CD0/1
  CL/1 -> Product1/1, Math Function/1
  Apolar (A2)/1 -> tune APolar/1
  Product/1 -> Sum1/2
  Apolar/1 -> "tune A1 "/1
  Product1/1 -> Sum1/3
  Math Function/1 -> Product/2
  tune APolar/1 -> Product/1

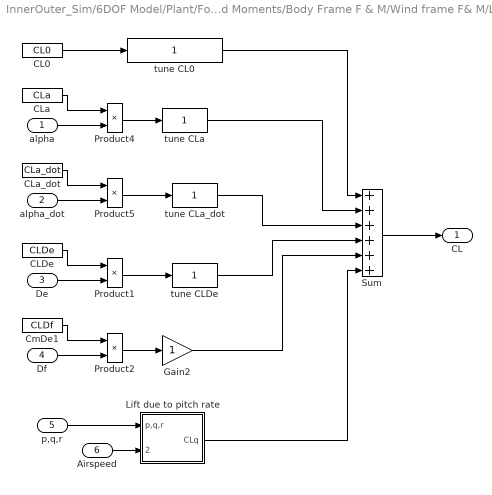
== system InnerOuter_Sim/6DOF Model/Plant/Forces and Moments/Body Frame F & M/Wind frame F& M/Longitudinal Channel/CL ==
  alpha : Inport
  alpha_dot : Inport  Port=2
  De : Inport  Port=3
  Df : Inport  Port=4
  p,q,r : Inport  Port=5
  Airspeed : Inport  Port=6
  CL0 : Constant  Value=CL0
  CLDe : Constant  Value=CLDe
  CLa : Constant  Value=CLa
  CLa_dot : Constant  Value=CLa_dot
  CmDe1 : Constant  Value=CLDf
  Gain2 : Gain  SaturateOnIntegerOverflow=on
  Lift due to pitch rate : Subsystem
  Product{1..2,4..5} (4 alike) : Product  SaturateOnIntegerOverflow=on
  Sum : Sum  Inputs=++++++  SaturateOnIntegerOverflow=on
  tune CL0 : simulink/Math Operations/Slider Gain  SystemSampleTime=-1  low=0  gain=1  high=2
  tune CLDe : simulink/Math Operations/Slider Gain  SystemSampleTime=-1  low=0  gain=1  high=200
  tune CLa : simulink/Math Operations/Slider Gain  SystemSampleTime=-1  low=0  gain=1  high=10
  tune CLa_dot : simulink/Math Operations/Slider Gain  SystemSampleTime=-1  low=0  gain=1  high=2
  CL : Outport
  wires:
  tune CLa/1 -> Sum/2
  CLa/1 -> Product4/1
  Product4/1 -> tune CLa/1
  alpha/1 -> Product4/2
  CLa_dot/1 -> Product5/1
  Product5/1 -> tune CLa_dot/1
  alpha_dot/1 -> Product5/2
  CLDe/1 -> Product1/1
  Product1/1 -> tune CLDe/1
  De/1 -> Product1/2
  Sum/1 -> CL/1
  Df/1 -> Product2/2
  Product2/1 -> Gain2/1
  CmDe1/1 -> Product2/1
  CL0/1 -> tune CL0/1
  tune CLa_dot/1 -> Sum/3
  tune CLDe/1 -> Sum/4
  Gain2/1 -> Sum/5
  Lift due to pitch rate/1(CLq) -> Sum/6
  p,q,r/1 -> Lift due to pitch rate/1(p,q,r)
  Airspeed/1 -> Lift due to pitch rate/2(Airspeed)
  tune CL0/1 -> Sum/1

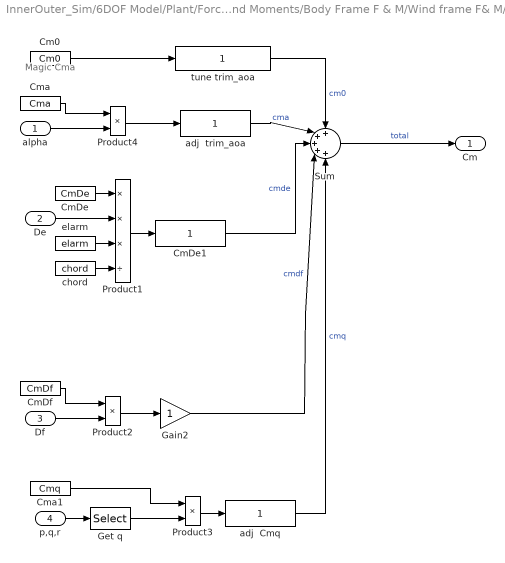
== system InnerOuter_Sim/6DOF Model/Plant/Forces and Moments/Body Frame F & M/Wind frame F& M/Longitudinal Channel/Cm ==
  note: Magic Cma
  alpha : Inport
  De : Inport  Port=2
  Df : Inport  Port=3
  p,q,r : Inport  Port=4
  Cm0 : Constant  Value=Cm0
  CmDe : Constant  Value=CmDe
  CmDe1 : simulink/Math Operations/Slider Gain  SystemSampleTime=-1  low=0  gain=1  high=3
  CmDf : Constant  Value=CmDf
  Cma : Constant  Value=Cma
  Cma1 : Constant  Value=Cmq
  Gain2 : Gain  SaturateOnIntegerOverflow=on
  Get q : Selector  IndexOptions=Index vector (dialog)  Indices=2  OutputSizes=[(-2)]  InputPortWidth=3
  Product1 : Product  Inputs=***/  SaturateOnIntegerOverflow=on
  Product2 : Product  SaturateOnIntegerOverflow=on
  Product3 : Product  SaturateOnIntegerOverflow=on
  Product4 : Product  SaturateOnIntegerOverflow=on
  Sum : Sum  Inputs=+++++  SaturateOnIntegerOverflow=on
  adj  Cmq : simulink/Math Operations/Slider Gain  SystemSampleTime=-1  low=0  gain=1  high=2
  adj  trim_aoa : simulink/Math Operations/Slider Gain  SystemSampleTime=-1  low=0  gain=1  high=2
  chord : Constant  Value=chord
  elarm : Constant  Value=elarm
  tune trim_aoa : simulink/Math Operations/Slider Gain  SystemSampleTime=-1  low=0  gain=1  high=1
  Cm : Outport
  wires:
  tune trim_aoa/1 -> Sum/1  "cm0"
  Gain2/1 -> Sum/4  "cmdf"
  CmDf/1 -> Product2/1
  Product2/1 -> Gain2/1
  Df/1 -> Product2/2
  Cma/1 -> Product4/1
  Product4/1 -> adj  trim_aoa/1
  alpha/1 -> Product4/2
  CmDe/1 -> Product1/1
  Product1/1 -> CmDe1/1
  De/1 -> Product1/2
  Sum/1 -> Cm/1  "total"
  adj  trim_aoa/1 -> Sum/2  "cma"
  Cm0/1 -> tune trim_aoa/1
  CmDe1/1 -> Sum/3  "cmde"
  Cma1/1 -> Product3/1
  Product3/1 -> adj  Cmq/1
  p,q,r/1 -> Get q/1
  adj  Cmq/1 -> Sum/5  "cmq"
  Get q/1 -> Product3/2
  elarm/1 -> Product1/3
  chord/1 -> Product1/4

== system InnerOuter_Sim/6DOF Model/Plant/Forces and Moments/Body Frame F & M/Wind frame F& M/Lateral Channel/Cl/roll factors ==
  p,q,r : Inport
  Airspeed : Inport  Port=2
  "Clp " : simulink/Math Operations/Slider Gain  SystemSampleTime=-1  low=0  gain=1  high=200
  "Clr " : simulink/Math Operations/Slider Gain  SystemSampleTime=-1  low=0  gain=1  high=50
  Constant : Constant  Value=Clp
  Constant1 : Constant  Value=Clr
  Get p : Selector  IndexOptions=Index vector (dialog)  Indices=1  OutputSizes=[(-2)]  InputPortWidth=3
  Get r : Selector  IndexOptions=Index vector (dialog)  Indices=3  OutputSizes=[(-2)]  InputPortWidth=3
  Product : Product  SaturateOnIntegerOverflow=on
  Product1 : Product  SaturateOnIntegerOverflow=on
  roll rate fact : Subsystem
  yaw rate fact : Subsystem
  Clp : Outport
  Clr : Outport  Port=2
  wires:
  Constant/1 -> "Clp "/1
  Constant1/1 -> "Clr "/1
  Product/1 -> Clp/1
  Product1/1 -> Clr/1
  "Clp "/1 -> Product/1
  roll rate fact/1(Roll Rate Fac) -> Product/2
  "Clr "/1 -> Product1/1
  yaw rate fact/1(Yaw Rate Fac) -> Product1/2
  Airspeed/1 -> roll rate fact/2(Airspeed), yaw rate fact/2(Airspeed)
  Get p/1 -> roll rate fact/1(p)
  p,q,r/1 -> Get p/1, Get r/1
  Get r/1 -> yaw rate fact/1(r)

== system InnerOuter_Sim/6DOF Model/Plant/Forces and Moments/Body Frame F & M/Wind frame F& M/Lateral Channel/Cn/yaw factors ==
  p,q,r : Inport
  Airspeed : Inport  Port=2
  Cnp1 : simulink/Math Operations/Slider Gain  SystemSampleTime=-1  low=-500  gain=1  high=50
  Cnr1 : simulink/Math Operations/Slider Gain  SystemSampleTime=-1  low=0  gain=1  high=500
  Constant : Constant  Value=Cnp
  Constant1 : Constant  Value=Cnr
  Get p : Selector  IndexOptions=Index vector (dialog)  Indices=1  OutputSizes=[(-2)]  InputPortWidth=3
  Get r : Selector  IndexOptions=Index vector (dialog)  Indices=3  OutputSizes=[(-2)]  InputPortWidth=3
  Product : Product  SaturateOnIntegerOverflow=on
  Product1 : Product  SaturateOnIntegerOverflow=on
  roll rate fact : Subsystem
  yaw rate fact : Subsystem
  Cnp : Outport
  Cnr : Outport  Port=2
  wires:
  Product/1 -> Cnp/1
  Product1/1 -> Cnr/1
  Constant1/1 -> Cnr1/1
  Cnr1/1 -> Product1/1
  yaw rate fact/1(Yaw Rate Fac) -> Product1/2
  Constant/1 -> Cnp1/1
  Cnp1/1 -> Product/1
  roll rate fact/1(Roll Rate Fac) -> Product/2
  Get p/1 -> roll rate fact/1(p)
  p,q,r/1 -> Get p/1, Get r/1
  Get r/1 -> yaw rate fact/1(r)
  Airspeed/1 -> roll rate fact/2(Airspeed), yaw rate fact/2(Airspeed)

== system InnerOuter_Sim/6DOF Model/Plant/Forces and Moments/Body Frame F & M/Wind frame F& M/Longitudinal Channel/CL/Lift due to pitch rate ==
  p,q,r : Inport
  Airspeed : Inport  Port=2
  Constant : Constant  Value=CLq
  Get q : Selector  IndexOptions=Index vector (dialog)  Indices=2  OutputSizes=[(-2)]  InputPortWidth=3
  Product : Product  SaturateOnIntegerOverflow=on
  pitch rate factor : Subsystem
  tune CLq : simulink/Math Operations/Slider Gain  SystemSampleTime=-1  low=0  gain=1  high=2000
  CLq : Outport
  wires:
  tune CLq/1 -> Product/1
  pitch rate factor/1(Pitch Rate Fac) -> Product/2
  Constant/1 -> tune CLq/1
  Product/1 -> CLq/1
  p,q,r/1 -> Get q/1
  Get q/1 -> pitch rate factor/1(q)
  Airspeed/1 -> pitch rate factor/2(Airspeed)

== system InnerOuter_Sim/6DOF Model/Plant/Forces and Moments/Body Frame F & M/Wind frame F& M/Lateral Channel/Cl/roll factors/roll rate fact ==
  p : Inport
  Airspeed : Inport  Port=2
  Cmq1 : Constant  Value=.5
  Cmq2 : Constant  Value=span
  Product : Product  Inputs=***/  SaturateOnIntegerOverflow=on
  Roll Rate Fac : Outport
  wires:
  Product/1 -> Roll Rate Fac/1
  p/1 -> Product/1
  Cmq1/1 -> Product/2
  Cmq2/1 -> Product/3
  Airspeed/1 -> Product/4

== system InnerOuter_Sim/6DOF Model/Plant/Forces and Moments/Body Frame F & M/Wind frame F& M/Lateral Channel/Cl/roll factors/yaw rate fact ==
  r : Inport
  Airspeed : Inport  Port=2
  Cmq1 : Constant  Value=.5
  Cmq2 : Constant  Value=span
  Product : Product  Inputs=***/  SaturateOnIntegerOverflow=on
  Yaw Rate Fac : Outport
  wires:
  r/1 -> Product/1
  Cmq1/1 -> Product/2
  Airspeed/1 -> Product/4
  Cmq2/1 -> Product/3
  Product/1 -> Yaw Rate Fac/1

== system InnerOuter_Sim/6DOF Model/Plant/Forces and Moments/Body Frame F & M/Wind frame F& M/Lateral Channel/Cn/yaw factors/roll rate fact ==
  p : Inport
  Airspeed : Inport  Port=2
  Cmq1 : Constant  Value=.5
  Cmq2 : Constant  Value=span
  Product : Product  Inputs=***/  SaturateOnIntegerOverflow=on
  Roll Rate Fac : Outport
  wires:
  Product/1 -> Roll Rate Fac/1
  p/1 -> Product/1
  Cmq1/1 -> Product/2
  Cmq2/1 -> Product/3
  Airspeed/1 -> Product/4

== system InnerOuter_Sim/6DOF Model/Plant/Forces and Moments/Body Frame F & M/Wind frame F& M/Lateral Channel/Cn/yaw factors/yaw rate fact ==
  r : Inport
  Airspeed : Inport  Port=2
  Cmq3 : Constant  Value=.5
  Cmq4 : Constant  Value=span
  Product1 : Product  Inputs=***/  SaturateOnIntegerOverflow=on
  Yaw Rate Fac : Outport
  wires:
  Product1/1 -> Yaw Rate Fac/1
  r/1 -> Product1/1
  Cmq3/1 -> Product1/2
  Cmq4/1 -> Product1/3
  Airspeed/1 -> Product1/4

== system InnerOuter_Sim/6DOF Model/Plant/Forces and Moments/Body Frame F & M/Wind frame F& M/Longitudinal Channel/CL/Lift due to pitch rate/pitch rate factor ==
  q : Inport
  Airspeed : Inport  Port=2
  Cmq2 : Constant  Value=chord
  Product : Product  Inputs=**/  SaturateOnIntegerOverflow=on
  Pitch Rate Fac : Outport
  wires:
  Product/1 -> Pitch Rate Fac/1
  q/1 -> Product/1
  Airspeed/1 -> Product/3
  Cmq2/1 -> Product/2

== matlab function 6DOF Model/Plant/Get GPS/Embedded MATLAB Function1 ==
  data: cog output inherited; Vn input inherited; Ve input inherited
function cog = getCOG(Vn, Ve)
% This block supports an embeddable subset of the MATLAB language.
% See the help menu for details. 

cog = atan2(Ve,Vn);
if cog < 0;
    cog = cog + 2*pi;
end
